simulink model "Ultrafiltration"  (R2025b)
settings: Solver=FixedStepAuto  StartTime=0.0  StopTime=1440  FixedStep=1  RelTol=1e-3
InitFcn:
  | initUF
  | tic;
StartFcn:
  | disp("Start...")
StopFcn:
  | disp("Stop...")
  | fprintf("SimTime: %.02f min", toc/60)
values from neighbouring files (symbols this model uses):
  BW_Max_Time = 90    [initUF.m]
  BW_Max_Vol_gal = 5000    [initUF.m]
  CEB_Max_Time = 1000    [initUF.m]
  CEB_Max_Vol_gal = 5000    [initUF.m]
  CIP_Max_Time = 15000    [initUF.m]
undefined symbols (not defined in the file or in its folder): LUT
libraries: simulink x30
(part 4 of 5)

== system Ultrafiltration/UF Maintenance Coordinator/arhive/UF_Operation State_7 ==
  UF7_MaintenanceStartSignal : Inport
  UF7_BeginStandby : Inport  Port=2
  UF7_BeginStartup : Inport  Port=3
  Bus Creator : BusCreator  Inputs=2
  Bus Selector : BusSelector  OutputSignals=UF_ShutdownCmd_7
  Bus Selector2 : BusSelector  OutputSignals=UF_StartupCmd_7
  Bus Selector7 : BusSelector  OutputSignals=UF_MaintCmd_7
  Delay Reset Signal : Memory
  Delay Startup : Memory
  UF7_Maintenance State : Stateflow chart  TreatAsAtomicUnit=on
  tag scope: UF7_MaintenanceRequest=global, UF7_MaintenanceState=global, UF7_OperatingState=global, UF7_StartupRequest=global
  wires:
  UF7_Maintenance State/1(unit_in_maint_queue) -> [UF7_MaintenanceRequest]  "UF7_MaintenanceRequestQueue"
  Bus Creator/1 -> [UF7_MaintenanceState]
  Delay Startup/1 -> [UF7_OperatingState], Bus Creator/1  "UF7_OperationsState"
  UF7_Maintenance State/4(maintenance_completion_indicator) -> Delay Reset Signal/1  "UF7_MaintenanceCompletionSignal"
  [UF7_Maintenance_Request] -> UF7_Maintenance State/2(maint_req)
  Delay Reset Signal/1 -> Bus Creator/2  "UF7_MaintenanceCompletionSignal"
  UF7_Maintenance State/3(unit_in_operation) -> Delay Startup/1  "UF7_OperationsState"
  UF7_Maintenance State/2(unit_in_startup_queue) -> [UF7_StartupRequest]  "UF7_StartupRequestQueue"
  UF7_BeginStandby/1 -> Bus Selector/1  "UF7_BeginStandby"
  Bus Selector/1 -> UF7_Maintenance State/3(standby_cmd)  "<UF_ShutdownCmd_7>"
  UF7_MaintenanceStartSignal/1 -> Bus Selector7/1  "UF7_MaintenanceStartSignal"
  Bus Selector7/1 -> UF7_Maintenance State/1(maint_cmd)  "<UF_MaintCmd_7>"
  UF7_BeginStartup/1 -> Bus Selector2/1  "UF7_BeginStartup"
  Bus Selector2/1 -> UF7_Maintenance State/4(startup_cmd)  "<UF_StartupCmd_7>"

== system Ultrafiltration/UF Maintenance Coordinator/arhive/UF_Operation State_8 ==
  UF8_MaintenanceStartSignal : Inport
  UF8_BeginStandby : Inport  Port=2
  UF8_BeginStartup : Inport  Port=3
  Bus Creator : BusCreator  Inputs=2
  Bus Selector : BusSelector  OutputSignals=UF_ShutdownCmd_8
  Bus Selector2 : BusSelector  OutputSignals=UF_StartupCmd_8
  Bus Selector8 : BusSelector  OutputSignals=UF_MaintCmd_8
  Delay Reset Signal : Memory
  Delay Startup : Memory
  UF8_Maintenance State : Stateflow chart  TreatAsAtomicUnit=on
  tag scope: UF8_MaintenanceRequest=global, UF8_MaintenanceState=global, UF8_OperatingState=global, UF8_StartupRequest=global
  wires:
  UF8_Maintenance State/1(unit_in_maint_queue) -> [UF8_MaintenanceRequest]  "UF8_MaintenanceRequestQueue"
  Bus Creator/1 -> [UF8_MaintenanceState]
  UF8_Maintenance State/4(maintenance_completion_indicator) -> Delay Reset Signal/1  "UF8_MaintenanceCompletionSignal"
  [UF8_Maintenance_Request] -> UF8_Maintenance State/2(maint_req)
  Delay Reset Signal/1 -> Bus Creator/2  "UF8_MaintenanceCompletionSignal"
  UF8_Maintenance State/3(unit_in_operation) -> Delay Startup/1  "UF8_OperationsState"
  UF8_Maintenance State/2(unit_in_startup_queue) -> [UF8_StartupRequest]  "UF8_StartupRequestQueue"
  UF8_BeginStandby/1 -> Bus Selector/1  "UF8_BeginStandby"
  Bus Selector/1 -> UF8_Maintenance State/3(standby_cmd)  "<UF_ShutdownCmd_8>"
  UF8_MaintenanceStartSignal/1 -> Bus Selector8/1  "UF8_MaintenanceStartSignal"
  Bus Selector8/1 -> UF8_Maintenance State/1(maint_cmd)  "<UF_MaintCmd_8>"
  UF8_BeginStartup/1 -> Bus Selector2/1  "UF8_BeginStartup"
  Bus Selector2/1 -> UF8_Maintenance State/4(startup_cmd)  "<UF_StartupCmd_8>"
  Delay Startup/1 -> [UF8_OperatingState], Bus Creator/1  "UF8_OperationsState"

== system Ultrafiltration/UF Maintenance Coordinator/arhive/UF_Operation State_9 ==
  UF9_MaintenanceStartSignal : Inport
  UF9_BeginStandby : Inport  Port=2
  UF9_BeginStartup : Inport  Port=3
  Bus Creator : BusCreator  Inputs=2
  Bus Selector : BusSelector  OutputSignals=UF_ShutdownCmd_9
  Bus Selector2 : BusSelector  OutputSignals=UF_StartupCmd_9
  Bus Selector9 : BusSelector  OutputSignals=UF_MaintCmd_9
  Delay Reset Signal : Memory
  Delay Startup : Memory
  UF9_Maintenance State : Stateflow chart  TreatAsAtomicUnit=on
  tag scope: UF9_MaintenanceRequest=global, UF9_MaintenanceState=global, UF9_OperatingState=global, UF9_StartupRequest=global
  wires:
  UF9_Maintenance State/1(unit_in_maint_queue) -> [UF9_MaintenanceRequest]  "UF9_MaintenanceRequestQueue"
  Bus Creator/1 -> [UF9_MaintenanceState]
  Delay Startup/1 -> [UF9_OperatingState], Bus Creator/1  "UF9_OperationsState"
  UF9_Maintenance State/4(maintenance_completion_indicator) -> Delay Reset Signal/1  "UF9_MaintenanceCompletionSignal"
  [UF9_Maintenance_Request] -> UF9_Maintenance State/2(maint_req)
  Delay Reset Signal/1 -> Bus Creator/2  "UF9_MaintenanceCompletionSignal"
  UF9_Maintenance State/3(unit_in_operation) -> Delay Startup/1  "UF9_OperationsState"
  UF9_Maintenance State/2(unit_in_startup_queue) -> [UF9_StartupRequest]  "UF9_StartupRequestQueue"
  UF9_BeginStandby/1 -> Bus Selector/1  "UF9_BeginStandby"
  Bus Selector/1 -> UF9_Maintenance State/3(standby_cmd)  "<UF_ShutdownCmd_9>"
  UF9_MaintenanceStartSignal/1 -> Bus Selector9/1  "UF9_MaintenanceStartSignal"
  Bus Selector9/1 -> UF9_Maintenance State/1(maint_cmd)  "<UF_MaintCmd_9>"
  UF9_BeginStartup/1 -> Bus Selector2/1  "UF9_BeginStartup"
  Bus Selector2/1 -> UF9_Maintenance State/4(startup_cmd)  "<UF_StartupCmd_9>"

== stateflow chart Ultrafiltration/UF Maintenance Coordinator/arhive/UF_Operation State_2/UF2_Maintenance State ==
  settings: sampleTime=1  executeAtInitialization=1
  note: Unit State Machine — FIFO Maintenance Dispatch
      | This chart controls a single filtration unit through four operational states: Standby, Running, Await_Maintenance, BW_Maintenance, and CEB_Maintenance.
      | The unit begins in Standby, awaiting a startup command from the central dispatcher. Once commanded on, it enters Running, where it operates normally and tracks cumulative downtime. If a maintenance request is triggered, the unit transitions to Await_Maintenance, remaining online until the dispatcher confirms it can be released.
      | Two maintenance sequences are supported. A Backwash (BW) is a fixed-duration event (4 timesteps). A Chemically Enhanced Backwash (CEB) is a stochastic event lasting between 30 and 90 timesteps, sampled from a uniform distribution at entry. CEB is always followed by a BW cycle.
      | Upon completion of maintenance, the unit returns to Standby and re-enters the startup queue at the back, consistent with FIFO dispatching logic.
  note: Unit_cmd = 1 for running, 0 for off.
  state Standby
    during:
    %Unit is off, but awaiting startup.
    unit_in_startup_queue = 1;
    unit_in_operation = 0;
    %Ensure that the maintenance resets are occuring.
    maintenance_completion_indicator = 0;
  state Running
    entry:
    %Reset downtime timer
    cycle_downtime = 0;
    during:
    %Unit on, not in maint queue.
    unit_in_operation = 1;
    unit_in_maint_queue = 0;
  state Await_standby
    %Unit , Enter maint Queue
    during:
    unit_in_operation = 0;
    unit_in_maint_queue = 1;
  state Await_maintenance
    %Unit stays on, Enter maint Queue
    during:
    unit_in_operation = 1;
    unit_in_maint_queue = 1;
  state CEB_Maintenance
    %Unit is in chemically enhanced backwash. After CEB, do BW.
    %At start, determine a maintenance time within a uniform range of 30-60 min.
    entry:
    needed_maint_time = 30 + (60-30) * rand();
    %Exit state when time in maintenance is >= expected time.
    during:
    unit_in_operation = -1; %unit in maintenance
    %update maintenance time every step.
    cycle_downtime = cycle_downtime + 1;
  state BW_Maintenance
    entry:
    needed_maint_time = 1.5;
    %Exit state when time in maintenance is >= expected time.
    during:
    unit_in_operation = -1; %unit in maintenance
    %update maintenance time every step.
    cycle_downtime = cycle_downtime + 1;
    %ensure that the CEB is not continually reseting.
    maintenance_completion_indicator = 0;
  note: Maintenance Completion Indicator represents a signal to reset the counters at the UF unit tracking backwash cycles (signal = 2) and time in operations (signal = 1). These are pulse signals that reset integrators.
  (default) -> Running
  Standby -> Running : [startup_cmd == 1]{unit_in_startup_queue = 0;}
  Running -> (junction 44) [order 2] : [standby_cmd == 1]
  Running -> Await_maintenance [order 1] : [maint_req ~=0]
  (junction 22) -> Standby
  Await_standby -> (junction 47) : [standby_cmd == 1 && maint_cmd == 1]
  (junction 47) -> (junction 11)
  (junction 44) -> Await_standby
  Await_maintenance -> (junction 11) [order 2] : [maint_req == 1 && maint_cmd == 1] {unit_in_maint_queue = 0;}
  (junction 11) -> BW_Maintenance
  Await_maintenance -> CEB_Maintenance [order 1] : [maint_req == 2 && maint_cmd ==1]
  CEB_Maintenance -> BW_Maintenance : [after(needed_maint_time, tick)]{maintenance_completion_indicator = 2;}
  BW_Maintenance -> (junction 22) : [after(needed_maint_time, tick)]
      | {maintenance_completion_indicator = 1;}
  data: maint_cmd input; maint_req input; standby_cmd input; startup_cmd input; unit_in_maint_queue output; unit_in_startup_queue output; cycle_downtime local; needed_maint_time local; unit_in_operation output; maintenance_completion_indicator output

== stateflow chart Ultrafiltration/UF Maintenance Coordinator/arhive/UF_Operation State_3/UF3_Maintenance State ==
  settings: sampleTime=1  executeAtInitialization=1
  note: Unit State Machine — FIFO Maintenance Dispatch
      | This chart controls a single filtration unit through four operational states: Standby, Running, Await_Maintenance, BW_Maintenance, and CEB_Maintenance.
      | The unit begins in Standby, awaiting a startup command from the central dispatcher. Once commanded on, it enters Running, where it operates normally and tracks cumulative downtime. If a maintenance request is triggered, the unit transitions to Await_Maintenance, remaining online until the dispatcher confirms it can be released.
      | Two maintenance sequences are supported. A Backwash (BW) is a fixed-duration event (4 timesteps). A Chemically Enhanced Backwash (CEB) is a stochastic event lasting between 30 and 90 timesteps, sampled from a uniform distribution at entry. CEB is always followed by a BW cycle.
      | Upon completion of maintenance, the unit returns to Standby and re-enters the startup queue at the back, consistent with FIFO dispatching logic.
  note: Unit_cmd = 1 for running, 0 for off.
  state Standby
    during:
    %Unit is off, but awaiting startup.
    unit_in_startup_queue = 1;
    unit_in_operation = 0;
    %Ensure that the maintenance resets are occuring.
    maintenance_completion_indicator = 0;
  state Running
    entry:
    %Reset downtime timer
    cycle_downtime = 0;
    during:
    %Unit on, not in maint queue.
    unit_in_operation = 1;
    unit_in_maint_queue = 0;
  state Await_standby
    %Unit , Enter maint Queue
    during:
    unit_in_operation = 0;
    unit_in_maint_queue = 1;
  state Await_maintenance
    %Unit stays on, Enter maint Queue
    during:
    unit_in_operation = 1;
    unit_in_maint_queue = 1;
  state CEB_Maintenance
    %Unit is in chemically enhanced backwash. After CEB, do BW.
    %At start, determine a maintenance time within a uniform range of 30-60 min.
    entry:
    needed_maint_time = 30 + (60-30) * rand();
    %Exit state when time in maintenance is >= expected time.
    during:
    unit_in_operation = -1; %unit in maintenance
    %update maintenance time every step.
    cycle_downtime = cycle_downtime + 1;
  state BW_Maintenance
    entry:
    needed_maint_time = 1.5;
    %Exit state when time in maintenance is >= expected time.
    during:
    unit_in_operation = -1; %unit in maintenance
    %update maintenance time every step.
    cycle_downtime = cycle_downtime + 1;
    %ensure that the CEB is not continually reseting.
    maintenance_completion_indicator = 0;
  note: Maintenance Completion Indicator represents a signal to reset the counters at the UF unit tracking backwash cycles (signal = 2) and time in operations (signal = 1). These are pulse signals that reset integrators.
  (default) -> Running
  Standby -> Running : [startup_cmd == 1]{unit_in_startup_queue = 0;}
  Running -> (junction 44) [order 2] : [standby_cmd == 1]
  Running -> Await_maintenance [order 1] : [maint_req ~=0]
  (junction 22) -> Standby
  Await_standby -> (junction 47) : [standby_cmd == 1 && maint_cmd == 1]
  (junction 47) -> (junction 11)
  (junction 44) -> Await_standby
  Await_maintenance -> (junction 11) [order 2] : [maint_req == 1 && maint_cmd == 1] {unit_in_maint_queue = 0;}
  (junction 11) -> BW_Maintenance
  Await_maintenance -> CEB_Maintenance [order 1] : [maint_req == 2 && maint_cmd ==1]
  CEB_Maintenance -> BW_Maintenance : [after(needed_maint_time, tick)]{maintenance_completion_indicator = 2;}
  BW_Maintenance -> (junction 22) : [after(needed_maint_time, tick)]
      | {maintenance_completion_indicator = 1;}
  data: maint_cmd input; maint_req input; standby_cmd input; startup_cmd input; unit_in_maint_queue output; unit_in_startup_queue output; cycle_downtime local; needed_maint_time local; unit_in_operation output; maintenance_completion_indicator output

== stateflow chart Ultrafiltration/UF Maintenance Coordinator/arhive/UF_Operation State_4/UF4_Maintenance State ==
  settings: sampleTime=1  executeAtInitialization=1
  note: Unit State Machine — FIFO Maintenance Dispatch
      | This chart controls a single filtration unit through four operational states: Standby, Running, Await_Maintenance, BW_Maintenance, and CEB_Maintenance.
      | The unit begins in Standby, awaiting a startup command from the central dispatcher. Once commanded on, it enters Running, where it operates normally and tracks cumulative downtime. If a maintenance request is triggered, the unit transitions to Await_Maintenance, remaining online until the dispatcher confirms it can be released.
      | Two maintenance sequences are supported. A Backwash (BW) is a fixed-duration event (4 timesteps). A Chemically Enhanced Backwash (CEB) is a stochastic event lasting between 30 and 90 timesteps, sampled from a uniform distribution at entry. CEB is always followed by a BW cycle.
      | Upon completion of maintenance, the unit returns to Standby and re-enters the startup queue at the back, consistent with FIFO dispatching logic.
  note: Unit_cmd = 1 for running, 0 for off.
  state Standby
    during:
    %Unit is off, but awaiting startup.
    unit_in_startup_queue = 1;
    unit_in_operation = 0;
    %Ensure that the maintenance resets are occuring.
    maintenance_completion_indicator = 0;
  state Running
    entry:
    %Reset downtime timer
    cycle_downtime = 0;
    during:
    %Unit on, not in maint queue.
    unit_in_operation = 1;
    unit_in_maint_queue = 0;
  state Await_standby
    %Unit , Enter maint Queue
    during:
    unit_in_operation = 0;
    unit_in_maint_queue = 1;
  state Await_maintenance
    %Unit stays on, Enter maint Queue
    during:
    unit_in_operation = 1;
    unit_in_maint_queue = 1;
  state CEB_Maintenance
    %Unit is in chemically enhanced backwash. After CEB, do BW.
    %At start, determine a maintenance time within a uniform range of 30-60 min.
    entry:
    needed_maint_time = 30 + (60-30) * rand();
    %Exit state when time in maintenance is >= expected time.
    during:
    unit_in_operation = -1; %unit in maintenance
    %update maintenance time every step.
    cycle_downtime = cycle_downtime + 1;
  state BW_Maintenance
    entry:
    needed_maint_time = 1.5;
    %Exit state when time in maintenance is >= expected time.
    during:
    unit_in_operation = -1; %unit in maintenance
    %update maintenance time every step.
    cycle_downtime = cycle_downtime + 1;
    %ensure that the CEB is not continually reseting.
    maintenance_completion_indicator = 0;
  note: Maintenance Completion Indicator represents a signal to reset the counters at the UF unit tracking backwash cycles (signal = 2) and time in operations (signal = 1). These are pulse signals that reset integrators.
  (default) -> Running
  Standby -> Running : [startup_cmd == 1]{unit_in_startup_queue = 0;}
  Running -> (junction 44) [order 2] : [standby_cmd == 1]
  Running -> Await_maintenance [order 1] : [maint_req ~=0]
  (junction 22) -> Standby
  Await_standby -> (junction 47) : [standby_cmd == 1 && maint_cmd == 1]
  (junction 47) -> (junction 11)
  (junction 44) -> Await_standby
  Await_maintenance -> (junction 11) [order 2] : [maint_req == 1 && maint_cmd == 1] {unit_in_maint_queue = 0;}
  (junction 11) -> BW_Maintenance
  Await_maintenance -> CEB_Maintenance [order 1] : [maint_req == 2 && maint_cmd ==1]
  CEB_Maintenance -> BW_Maintenance : [after(needed_maint_time, tick)]{maintenance_completion_indicator = 2;}
  BW_Maintenance -> (junction 22) : [after(needed_maint_time, tick)]
      | {maintenance_completion_indicator = 1;}
  data: maint_cmd input; maint_req input; standby_cmd input; startup_cmd input; unit_in_maint_queue output; unit_in_startup_queue output; cycle_downtime local; needed_maint_time local; unit_in_operation output; maintenance_completion_indicator output

== stateflow chart Ultrafiltration/UF Maintenance Coordinator/arhive/UF_Operation State_5/UF5_Maintenance State ==
  settings: sampleTime=1  executeAtInitialization=1
  note: Unit State Machine — FIFO Maintenance Dispatch
      | This chart controls a single filtration unit through four operational states: Standby, Running, Await_Maintenance, BW_Maintenance, and CEB_Maintenance.
      | The unit begins in Standby, awaiting a startup command from the central dispatcher. Once commanded on, it enters Running, where it operates normally and tracks cumulative downtime. If a maintenance request is triggered, the unit transitions to Await_Maintenance, remaining online until the dispatcher confirms it can be released.
      | Two maintenance sequences are supported. A Backwash (BW) is a fixed-duration event (4 timesteps). A Chemically Enhanced Backwash (CEB) is a stochastic event lasting between 30 and 90 timesteps, sampled from a uniform distribution at entry. CEB is always followed by a BW cycle.
      | Upon completion of maintenance, the unit returns to Standby and re-enters the startup queue at the back, consistent with FIFO dispatching logic.
  note: Unit_cmd = 1 for running, 0 for off.
  state Standby
    during:
    %Unit is off, but awaiting startup.
    unit_in_startup_queue = 1;
    unit_in_operation = 0;
    %Ensure that the maintenance resets are occuring.
    maintenance_completion_indicator = 0;
  state Running
    entry:
    %Reset downtime timer
    cycle_downtime = 0;
    during:
    %Unit on, not in maint queue.
    unit_in_operation = 1;
    unit_in_maint_queue = 0;
  state Await_standby
    %Unit , Enter maint Queue
    during:
    unit_in_operation = 0;
    unit_in_maint_queue = 1;
  state Await_maintenance
    %Unit stays on, Enter maint Queue
    during:
    unit_in_operation = 1;
    unit_in_maint_queue = 1;
  state CEB_Maintenance
    %Unit is in chemically enhanced backwash. After CEB, do BW.
    %At start, determine a maintenance time within a uniform range of 30-60 min.
    entry:
    needed_maint_time = 30 + (60-30) * rand();
    %Exit state when time in maintenance is >= expected time.
    during:
    unit_in_operation = -1; %unit in maintenance
    %update maintenance time every step.
    cycle_downtime = cycle_downtime + 1;
  state BW_Maintenance
    entry:
    needed_maint_time = 1.5;
    %Exit state when time in maintenance is >= expected time.
    during:
    unit_in_operation = -1; %unit in maintenance
    %update maintenance time every step.
    cycle_downtime = cycle_downtime + 1;
    %ensure that the CEB is not continually reseting.
    maintenance_completion_indicator = 0;
  note: Maintenance Completion Indicator represents a signal to reset the counters at the UF unit tracking backwash cycles (signal = 2) and time in operations (signal = 1). These are pulse signals that reset integrators.
  (default) -> Running
  Standby -> Running : [startup_cmd == 1]{unit_in_startup_queue = 0;}
  Running -> (junction 44) [order 2] : [standby_cmd == 1]
  Running -> Await_maintenance [order 1] : [maint_req ~=0]
  (junction 22) -> Standby
  Await_standby -> (junction 47) : [standby_cmd == 1 && maint_cmd == 1]
  (junction 47) -> (junction 11)
  (junction 44) -> Await_standby
  Await_maintenance -> (junction 11) [order 2] : [maint_req == 1 && maint_cmd == 1] {unit_in_maint_queue = 0;}
  (junction 11) -> BW_Maintenance
  Await_maintenance -> CEB_Maintenance [order 1] : [maint_req == 2 && maint_cmd ==1]
  CEB_Maintenance -> BW_Maintenance : [after(needed_maint_time, tick)]{maintenance_completion_indicator = 2;}
  BW_Maintenance -> (junction 22) : [after(needed_maint_time, tick)]
      | {maintenance_completion_indicator = 1;}
  data: maint_cmd input; maint_req input; standby_cmd input; startup_cmd input; unit_in_maint_queue output; unit_in_startup_queue output; cycle_downtime local; needed_maint_time local; unit_in_operation output; maintenance_completion_indicator output

== stateflow chart Ultrafiltration/UF Maintenance Coordinator/arhive/UF_Operation State_6/UF6_Maintenance State ==
  settings: sampleTime=1  executeAtInitialization=1
  note: Unit State Machine — FIFO Maintenance Dispatch
      | This chart controls a single filtration unit through four operational states: Standby, Running, Await_Maintenance, BW_Maintenance, and CEB_Maintenance.
      | The unit begins in Standby, awaiting a startup command from the central dispatcher. Once commanded on, it enters Running, where it operates normally and tracks cumulative downtime. If a maintenance request is triggered, the unit transitions to Await_Maintenance, remaining online until the dispatcher confirms it can be released.
      | Two maintenance sequences are supported. A Backwash (BW) is a fixed-duration event (4 timesteps). A Chemically Enhanced Backwash (CEB) is a stochastic event lasting between 30 and 90 timesteps, sampled from a uniform distribution at entry. CEB is always followed by a BW cycle.
      | Upon completion of maintenance, the unit returns to Standby and re-enters the startup queue at the back, consistent with FIFO dispatching logic.
  note: Unit_cmd = 1 for running, 0 for off.
  state Standby
    during:
    %Unit is off, but awaiting startup.
    unit_in_startup_queue = 1;
    unit_in_operation = 0;
    %Ensure that the maintenance resets are occuring.
    maintenance_completion_indicator = 0;
  state Running
    entry:
    %Reset downtime timer
    cycle_downtime = 0;
    during:
    %Unit on, not in maint queue.
    unit_in_operation = 1;
    unit_in_maint_queue = 0;
  state Await_standby
    %Unit , Enter maint Queue
    during:
    unit_in_operation = 0;
    unit_in_maint_queue = 1;
  state Await_maintenance
    %Unit stays on, Enter maint Queue
    during:
    unit_in_operation = 1;
    unit_in_maint_queue = 1;
  state CEB_Maintenance
    %Unit is in chemically enhanced backwash. After CEB, do BW.
    %At start, determine a maintenance time within a uniform range of 30-60 min.
    entry:
    needed_maint_time = 30 + (60-30) * rand();
    %Exit state when time in maintenance is >= expected time.
    during:
    unit_in_operation = -1; %unit in maintenance
    %update maintenance time every step.
    cycle_downtime = cycle_downtime + 1;
  state BW_Maintenance
    entry:
    needed_maint_time = 1.5;
    %Exit state when time in maintenance is >= expected time.
    during:
    unit_in_operation = -1; %unit in maintenance
    %update maintenance time every step.
    cycle_downtime = cycle_downtime + 1;
    %ensure that the CEB is not continually reseting.
    maintenance_completion_indicator = 0;
  note: Maintenance Completion Indicator represents a signal to reset the counters at the UF unit tracking backwash cycles (signal = 2) and time in operations (signal = 1). These are pulse signals that reset integrators.
  (default) -> Running
  Standby -> Running : [startup_cmd == 1]{unit_in_startup_queue = 0;}
  Running -> (junction 44) [order 2] : [standby_cmd == 1]
  Running -> Await_maintenance [order 1] : [maint_req ~=0]
  (junction 22) -> Standby
  Await_standby -> (junction 47) : [standby_cmd == 1 && maint_cmd == 1]
  (junction 47) -> (junction 11)
  (junction 44) -> Await_standby
  Await_maintenance -> (junction 11) [order 2] : [maint_req == 1 && maint_cmd == 1] {unit_in_maint_queue = 0;}
  (junction 11) -> BW_Maintenance
  Await_maintenance -> CEB_Maintenance [order 1] : [maint_req == 2 && maint_cmd ==1]
  CEB_Maintenance -> BW_Maintenance : [after(needed_maint_time, tick)]{maintenance_completion_indicator = 2;}
  BW_Maintenance -> (junction 22) : [after(needed_maint_time, tick)]
      | {maintenance_completion_indicator = 1;}
  data: maint_cmd input; maint_req input; standby_cmd input; startup_cmd input; unit_in_maint_queue output; unit_in_startup_queue output; cycle_downtime local; needed_maint_time local; unit_in_operation output; maintenance_completion_indicator output

== stateflow chart Ultrafiltration/UF Maintenance Coordinator/arhive/UF_Operation State_7/UF7_Maintenance State ==
  settings: sampleTime=1  executeAtInitialization=1
  note: Unit State Machine — FIFO Maintenance Dispatch
      | This chart controls a single filtration unit through four operational states: Standby, Running, Await_Maintenance, BW_Maintenance, and CEB_Maintenance.
      | The unit begins in Standby, awaiting a startup command from the central dispatcher. Once commanded on, it enters Running, where it operates normally and tracks cumulative downtime. If a maintenance request is triggered, the unit transitions to Await_Maintenance, remaining online until the dispatcher confirms it can be released.
      | Two maintenance sequences are supported. A Backwash (BW) is a fixed-duration event (4 timesteps). A Chemically Enhanced Backwash (CEB) is a stochastic event lasting between 30 and 90 timesteps, sampled from a uniform distribution at entry. CEB is always followed by a BW cycle.
      | Upon completion of maintenance, the unit returns to Standby and re-enters the startup queue at the back, consistent with FIFO dispatching logic.
  note: Unit_cmd = 1 for running, 0 for off.
  state Standby
    during:
    %Unit is off, but awaiting startup.
    unit_in_startup_queue = 1;
    unit_in_operation = 0;
    %Ensure that the maintenance resets are occuring.
    maintenance_completion_indicator = 0;
  state Running
    entry:
    %Reset downtime timer
    cycle_downtime = 0;
    during:
    %Unit on, not in maint queue.
    unit_in_operation = 1;
    unit_in_maint_queue = 0;
  state Await_standby
    %Unit , Enter maint Queue
    during:
    unit_in_operation = 0;
    unit_in_maint_queue = 1;
  state Await_maintenance
    %Unit stays on, Enter maint Queue
    during:
    unit_in_operation = 1;
    unit_in_maint_queue = 1;
  state CEB_Maintenance
    %Unit is in chemically enhanced backwash. After CEB, do BW.
    %At start, determine a maintenance time within a uniform range of 30-60 min.
    entry:
    needed_maint_time = 30 + (60-30) * rand();
    %Exit state when time in maintenance is >= expected time.
    during:
    unit_in_operation = -1; %unit in maintenance
    %update maintenance time every step.
    cycle_downtime = cycle_downtime + 1;
  state BW_Maintenance
    entry:
    needed_maint_time = 1.5;
    %Exit state when time in maintenance is >= expected time.
    during:
    unit_in_operation = -1; %unit in maintenance
    %update maintenance time every step.
    cycle_downtime = cycle_downtime + 1;
    %ensure that the CEB is not continually reseting.
    maintenance_completion_indicator = 0;
  note: Maintenance Completion Indicator represents a signal to reset the counters at the UF unit tracking backwash cycles (signal = 2) and time in operations (signal = 1). These are pulse signals that reset integrators.
  (default) -> Running
  Standby -> Running : [startup_cmd == 1]{unit_in_startup_queue = 0;}
  Running -> (junction 44) [order 2] : [standby_cmd == 1]
  Running -> Await_maintenance [order 1] : [maint_req ~=0]
  (junction 22) -> Standby
  Await_standby -> (junction 47) : [standby_cmd == 1 && maint_cmd == 1]
  (junction 47) -> (junction 11)
  (junction 44) -> Await_standby
  Await_maintenance -> (junction 11) [order 2] : [maint_req == 1 && maint_cmd == 1] {unit_in_maint_queue = 0;}
  (junction 11) -> BW_Maintenance
  Await_maintenance -> CEB_Maintenance [order 1] : [maint_req == 2 && maint_cmd ==1]
  CEB_Maintenance -> BW_Maintenance : [after(needed_maint_time, tick)]{maintenance_completion_indicator = 2;}
  BW_Maintenance -> (junction 22) : [after(needed_maint_time, tick)]
      | {maintenance_completion_indicator = 1;}
  data: maint_cmd input; maint_req input; standby_cmd input; startup_cmd input; unit_in_maint_queue output; unit_in_startup_queue output; cycle_downtime local; needed_maint_time local; unit_in_operation output; maintenance_completion_indicator output

== stateflow chart Ultrafiltration/UF Maintenance Coordinator/arhive/UF_Operation State_8/UF8_Maintenance State ==
  settings: sampleTime=1  executeAtInitialization=1
  note: Unit State Machine — FIFO Maintenance Dispatch
      | This chart controls a single filtration unit through four operational states: Standby, Running, Await_Maintenance, BW_Maintenance, and CEB_Maintenance.
      | The unit begins in Standby, awaiting a startup command from the central dispatcher. Once commanded on, it enters Running, where it operates normally and tracks cumulative downtime. If a maintenance request is triggered, the unit transitions to Await_Maintenance, remaining online until the dispatcher confirms it can be released.
      | Two maintenance sequences are supported. A Backwash (BW) is a fixed-duration event (4 timesteps). A Chemically Enhanced Backwash (CEB) is a stochastic event lasting between 30 and 90 timesteps, sampled from a uniform distribution at entry. CEB is always followed by a BW cycle.
      | Upon completion of maintenance, the unit returns to Standby and re-enters the startup queue at the back, consistent with FIFO dispatching logic.
  note: Unit_cmd = 1 for running, 0 for off.
  state Standby
    during:
    %Unit is off, but awaiting startup.
    unit_in_startup_queue = 1;
    unit_in_operation = 0;
    %Ensure that the maintenance resets are occuring.
    maintenance_completion_indicator = 0;
  state Running
    entry:
    %Reset downtime timer
    cycle_downtime = 0;
    during:
    %Unit on, not in maint queue.
    unit_in_operation = 1;
    unit_in_maint_queue = 0;
  state Await_standby
    %Unit , Enter maint Queue
    during:
    unit_in_operation = 0;
    unit_in_maint_queue = 1;
  state Await_maintenance
    %Unit stays on, Enter maint Queue
    during:
    unit_in_operation = 1;
    unit_in_maint_queue = 1;
  state CEB_Maintenance
    %Unit is in chemically enhanced backwash. After CEB, do BW.
    %At start, determine a maintenance time within a uniform range of 30-60 min.
    entry:
    needed_maint_time = 30 + (60-30) * rand();
    %Exit state when time in maintenance is >= expected time.
    during:
    unit_in_operation = -1; %unit in maintenance
    %update maintenance time every step.
    cycle_downtime = cycle_downtime + 1;
  state BW_Maintenance
    entry:
    needed_maint_time = 1.5;
    %Exit state when time in maintenance is >= expected time.
    during:
    unit_in_operation = -1; %unit in maintenance
    %update maintenance time every step.
    cycle_downtime = cycle_downtime + 1;
    %ensure that the CEB is not continually reseting.
    maintenance_completion_indicator = 0;
  note: Maintenance Completion Indicator represents a signal to reset the counters at the UF unit tracking backwash cycles (signal = 2) and time in operations (signal = 1). These are pulse signals that reset integrators.
  (default) -> Running
  Standby -> Running : [startup_cmd == 1]{unit_in_startup_queue = 0;}
  Running -> (junction 44) [order 2] : [standby_cmd == 1]
  Running -> Await_maintenance [order 1] : [maint_req ~=0]
  (junction 22) -> Standby
  Await_standby -> (junction 47) : [standby_cmd == 1 && maint_cmd == 1]
  (junction 47) -> (junction 11)
  (junction 44) -> Await_standby
  Await_maintenance -> (junction 11) [order 2] : [maint_req == 1 && maint_cmd == 1] {unit_in_maint_queue = 0;}
  (junction 11) -> BW_Maintenance
  Await_maintenance -> CEB_Maintenance [order 1] : [maint_req == 2 && maint_cmd ==1]
  CEB_Maintenance -> BW_Maintenance : [after(needed_maint_time, tick)]{maintenance_completion_indicator = 2;}
  BW_Maintenance -> (junction 22) : [after(needed_maint_time, tick)]
      | {maintenance_completion_indicator = 1;}
  data: maint_cmd input; maint_req input; standby_cmd input; startup_cmd input; unit_in_maint_queue output; unit_in_startup_queue output; cycle_downtime local; needed_maint_time local; unit_in_operation output; maintenance_completion_indicator output

== stateflow chart Ultrafiltration/UF Maintenance Coordinator/arhive/UF_Operation State_9/UF9_Maintenance State ==
  settings: sampleTime=1  executeAtInitialization=1
  note: Unit State Machine — FIFO Maintenance Dispatch
      | This chart controls a single filtration unit through four operational states: Standby, Running, Await_Maintenance, BW_Maintenance, and CEB_Maintenance.
      | The unit begins in Standby, awaiting a startup command from the central dispatcher. Once commanded on, it enters Running, where it operates normally and tracks cumulative downtime. If a maintenance request is triggered, the unit transitions to Await_Maintenance, remaining online until the dispatcher confirms it can be released.
      | Two maintenance sequences are supported. A Backwash (BW) is a fixed-duration event (4 timesteps). A Chemically Enhanced Backwash (CEB) is a stochastic event lasting between 30 and 90 timesteps, sampled from a uniform distribution at entry. CEB is always followed by a BW cycle.
      | Upon completion of maintenance, the unit returns to Standby and re-enters the startup queue at the back, consistent with FIFO dispatching logic.
  note: Unit_cmd = 1 for running, 0 for off.
  state Standby
    during:
    %Unit is off, but awaiting startup.
    unit_in_startup_queue = 1;
    unit_in_operation = 0;
    %Ensure that the maintenance resets are occuring.
    maintenance_completion_indicator = 0;
  state Running
    entry:
    %Reset downtime timer
    cycle_downtime = 0;
    during:
    %Unit on, not in maint queue.
    unit_in_operation = 1;
    unit_in_maint_queue = 0;
  state Await_standby
    %Unit , Enter maint Queue
    during:
    unit_in_operation = 0;
    unit_in_maint_queue = 1;
  state Await_maintenance
    %Unit stays on, Enter maint Queue
    during:
    unit_in_operation = 1;
    unit_in_maint_queue = 1;
  state CEB_Maintenance
    %Unit is in chemically enhanced backwash. After CEB, do BW.
    %At start, determine a maintenance time within a uniform range of 30-60 min.
    entry:
    needed_maint_time = 30 + (60-30) * rand();
    %Exit state when time in maintenance is >= expected time.
    during:
    unit_in_operation = -1; %unit in maintenance
    %update maintenance time every step.
    cycle_downtime = cycle_downtime + 1;
  state BW_Maintenance
    entry:
    needed_maint_time = 1.5;
    %Exit state when time in maintenance is >= expected time.
    during:
    unit_in_operation = -1; %unit in maintenance
    %update maintenance time every step.
    cycle_downtime = cycle_downtime + 1;
    %ensure that the CEB is not continually reseting.
    maintenance_completion_indicator = 0;
  note: Maintenance Completion Indicator represents a signal to reset the counters at the UF unit tracking backwash cycles (signal = 2) and time in operations (signal = 1). These are pulse signals that reset integrators.
  (default) -> Running
  Standby -> Running : [startup_cmd == 1]{unit_in_startup_queue = 0;}
  Running -> (junction 44) [order 2] : [standby_cmd == 1]
  Running -> Await_maintenance [order 1] : [maint_req ~=0]
  (junction 22) -> Standby
  Await_standby -> (junction 47) : [standby_cmd == 1 && maint_cmd == 1]
  (junction 47) -> (junction 11)
  (junction 44) -> Await_standby
  Await_maintenance -> (junction 11) [order 2] : [maint_req == 1 && maint_cmd == 1] {unit_in_maint_queue = 0;}
  (junction 11) -> BW_Maintenance
  Await_maintenance -> CEB_Maintenance [order 1] : [maint_req == 2 && maint_cmd ==1]
  CEB_Maintenance -> BW_Maintenance : [after(needed_maint_time, tick)]{maintenance_completion_indicator = 2;}
  BW_Maintenance -> (junction 22) : [after(needed_maint_time, tick)]
      | {maintenance_completion_indicator = 1;}
  data: maint_cmd input; maint_req input; standby_cmd input; startup_cmd input; unit_in_maint_queue output; unit_in_startup_queue output; cycle_downtime local; needed_maint_time local; unit_in_operation output; maintenance_completion_indicator output

== stateflow chart Ultrafiltration/UF Maintenance Coordinator/arhive/UF_Operation State_10/UF10_Maintenance State ==
  settings: sampleTime=1  executeAtInitialization=1
  note: Unit State Machine — FIFO Maintenance Dispatch
      | This chart controls a single filtration unit through four operational states: Standby, Running, Await_Maintenance, BW_Maintenance, and CEB_Maintenance.
      | The unit begins in Standby, awaiting a startup command from the central dispatcher. Once commanded on, it enters Running, where it operates normally and tracks cumulative downtime. If a maintenance request is triggered, the unit transitions to Await_Maintenance, remaining online until the dispatcher confirms it can be released.
      | Two maintenance sequences are supported. A Backwash (BW) is a fixed-duration event (4 timesteps). A Chemically Enhanced Backwash (CEB) is a stochastic event lasting between 30 and 90 timesteps, sampled from a uniform distribution at entry. CEB is always followed by a BW cycle.
      | Upon completion of maintenance, the unit returns to Standby and re-enters the startup queue at the back, consistent with FIFO dispatching logic.
  note: Unit_cmd = 1 for running, 0 for off.
  state Standby
    during:
    %Unit is off, but awaiting startup.
    unit_in_startup_queue = 1;
    unit_in_operation = 0;
    %Ensure that the maintenance resets are occuring.
    maintenance_completion_indicator = 0;
  state Running
    entry:
    %Reset downtime timer
    cycle_downtime = 0;
    during:
    %Unit on, not in maint queue.
    unit_in_operation = 1;
    unit_in_maint_queue = 0;
  state Await_standby
    %Unit , Enter maint Queue
    during:
    unit_in_operation = 0;
    unit_in_maint_queue = 1;
  state Await_maintenance
    %Unit stays on, Enter maint Queue
    during:
    unit_in_operation = 1;
    unit_in_maint_queue = 1;
  state CEB_Maintenance
    %Unit is in chemically enhanced backwash. After CEB, do BW.
    %At start, determine a maintenance time within a uniform range of 30-60 min.
    entry:
    needed_maint_time = 30 + (60-30) * rand();
    %Exit state when time in maintenance is >= expected time.
    during:
    unit_in_operation = -1; %unit in maintenance
    %update maintenance time every step.
    cycle_downtime = cycle_downtime + 1;
  state BW_Maintenance
    entry:
    needed_maint_time = 1.5;
    %Exit state when time in maintenance is >= expected time.
    during:
    unit_in_operation = -1; %unit in maintenance
    %update maintenance time every step.
    cycle_downtime = cycle_downtime + 1;
    %ensure that the CEB is not continually reseting.
    maintenance_completion_indicator = 0;
  note: Maintenance Completion Indicator represents a signal to reset the counters at the UF unit tracking backwash cycles (signal = 2) and time in operations (signal = 1). These are pulse signals that reset integrators.
  (default) -> Running
  Standby -> Running : [startup_cmd == 1]{unit_in_startup_queue = 0;}
  Running -> (junction 44) [order 2] : [standby_cmd == 1]
  Running -> Await_maintenance [order 1] : [maint_req ~=0]
  (junction 22) -> Standby
  Await_standby -> (junction 47) : [standby_cmd == 1 && maint_cmd == 1]
  (junction 47) -> (junction 11)
  (junction 44) -> Await_standby
  Await_maintenance -> (junction 11) [order 2] : [maint_req == 1 && maint_cmd == 1] {unit_in_maint_queue = 0;}
  (junction 11) -> BW_Maintenance
  Await_maintenance -> CEB_Maintenance [order 1] : [maint_req == 2 && maint_cmd ==1]
  CEB_Maintenance -> BW_Maintenance : [after(needed_maint_time, tick)]{maintenance_completion_indicator = 2;}
  BW_Maintenance -> (junction 22) : [after(needed_maint_time, tick)]
      | {maintenance_completion_indicator = 1;}
  data: maint_cmd input; maint_req input; standby_cmd input; startup_cmd input; unit_in_maint_queue output; unit_in_startup_queue output; cycle_downtime local; needed_maint_time local; unit_in_operation output; maintenance_completion_indicator output

== stateflow chart Ultrafiltration/UF Maintenance Coordinator/Sample_Stateflows ==
  settings: sampleTime=1  executeAtInitialization=1
  note: Unit State Machine — FIFO Maintenance Dispatch
      | This chart controls a single filtration unit through four operational states: Standby, Running, Await_Maintenance, BW_Maintenance, and CEB_Maintenance.
      | The unit begins in Standby, awaiting a startup command from the central dispatcher. Once commanded on, it enters Running, where it operates normally and tracks cumulative downtime. If a maintenance request is triggered, the unit transitions to Await_Maintenance, remaining online until the dispatcher confirms it can be released.
      | Two maintenance sequences are supported. A Backwash (BW) is a fixed-duration event (4 timesteps). A Chemically Enhanced Backwash (CEB) is a stochastic event lasting between 30 and 90 timesteps, sampled from a uniform distribution at entry. CEB is always followed by a BW cycle.
      | Upon completion of maintenance, the unit returns to Standby and re-enters the startup queue at the back, consistent with FIFO dispatching logic.
  note: Unit_cmd = 1 for running, 0 for off.
  state Standby
    during:
    %Unit is off, but awaiting startup.
    unit_in_startup_queue = 1;
    unit_in_operation = 0;
    %Ensure that the maintenance resets are occuring.
    maintenance_completion_indicator = 0;
  state Running
    entry:
    %Reset downtime timer
    cycle_downtime = 0;
    during:
    %Unit on, not in maint queue.
    unit_in_operation = 1;
    unit_in_maint_queue = 0;
  state Await_standby
    %Unit , Enter maint Queue
    during:
    unit_in_operation = 0;
    unit_in_maint_queue = 1;
  state Await_maintenance
    %Unit stays on, Enter maint Queue
    during:
    unit_in_operation = 1;
    unit_in_maint_queue = 1;
  state CEB_Maintenance
    %Unit is in chemically enhanced backwash. After CEB, do BW.
    %At start, determine a maintenance time within a uniform range of 30-60 min.
    entry:
    needed_maint_time = 30 + (60-30) * rand();
    %Exit state when time in maintenance is >= expected time.
    during:
    unit_in_operation = -1; %unit in maintenance
    %update maintenance time every step.
    cycle_downtime = cycle_downtime + 1;
  state BW_Maintenance
    entry:
    needed_maint_time = 1.5;
    %Exit state when time in maintenance is >= expected time.
    during:
    unit_in_operation = -1; %unit in maintenance
    %update maintenance time every step.
    cycle_downtime = cycle_downtime + 1;
    %ensure that the CEB is not continually reseting.
    maintenance_completion_indicator = 0;
  note: Maintenance Completion Indicator represents a signal to reset the counters at the UF unit tracking backwash cycles (signal = 2) and time in operations (signal = 1). These are pulse signals that reset integrators.
  (default) -> Running
  Standby -> Running : [startup_cmd == 1]{unit_in_startup_queue = 0;}
  Running -> (junction 44) [order 2] : [standby_cmd == 1]
  Running -> Await_maintenance [order 1] : [maint_req ~=0]
  (junction 22) -> Standby
  Await_standby -> (junction 47) : [standby_cmd == 1 && maint_cmd == 1]
  (junction 47) -> (junction 11)
  (junction 44) -> Await_standby
  Await_maintenance -> (junction 11) [order 2] : [maint_req == 1 && maint_cmd == 1] {unit_in_maint_queue = 0;}
  (junction 11) -> BW_Maintenance
  Await_maintenance -> CEB_Maintenance [order 1] : [maint_req == 2 && maint_cmd ==1]
  CEB_Maintenance -> BW_Maintenance : [after(needed_maint_time, tick)]{maintenance_completion_indicator = 2;}
  BW_Maintenance -> (junction 22) : [after(needed_maint_time, tick)]
      | {maintenance_completion_indicator = 1;}
  data: maint_cmd input; maint_req input; standby_cmd input; startup_cmd input; unit_in_maint_queue output; unit_in_startup_queue output; cycle_downtime local; needed_maint_time local; unit_in_operation output; maintenance_completion_indicator output
